simulink model "NLGuidance_12B_with_contracts_PP"  (R2019b)
settings: Solver=FixedStepDiscrete  StartTime=0.0  StopTime=10.0  FixedStep=0.020000  RelTol=1e-3  EnableMultiTasking=on
model workspace (MAT data in the model file):
  ContractValidatorBlocksMap = containers.Map
  ContractValidatorBlocksMap.serialization.keys = {'NLGuidance_12B/contract/validator', 'NLGuidance_12B_with_contracts/contract/validator'}
  ContractValidatorBlocksMap.serialization.values{1}.block = 'NLGuidance_12B/contract/validator'
  ContractValidatorBlocksMap.serialization.values{1}.assumePorts = 2
  ContractValidatorBlocksMap.serialization.values{1}.guaranteePorts = 6
  ContractValidatorBlocksMap.serialization.values{1}.modeBlocksPorts = 0
  ContractValidatorBlocksMap.serialization.values{1}.portHandles.Inport = [1044.00036621 1045.00036621 1046.00036621 1047.00036621 1048.00036621 1049.00036621 1050.00036621 1051.00036621]
  ContractValidatorBlocksMap.serialization.values{1}.portHandles.Outport = 1052.00036621
  ContractValidatorBlocksMap.serialization.values{1}.portHandles.Enable = []
  ContractValidatorBlocksMap.serialization.values{1}.portHandles.Trigger = []
  ContractValidatorBlocksMap.serialization.values{1}.portHandles.State = []
  ContractValidatorBlocksMap.serialization.values{1}.portHandles.LConn = []
  ContractValidatorBlocksMap.serialization.values{1}.portHandles.RConn = []
  ContractValidatorBlocksMap.serialization.values{1}.portHandles.Ifaction = []
  ContractValidatorBlocksMap.serialization.values{1}.portHandles.Reset = []
  ContractValidatorBlocksMap.serialization.values{1}.portConnectivity(1).Type = '1'
  ContractValidatorBlocksMap.serialization.values{1}.portConnectivity(1).Position = [365 -130]
  ContractValidatorBlocksMap.serialization.values{1}.portConnectivity(1).SrcBlock = 945.000488281
  ContractValidatorBlocksMap.serialization.values{1}.portConnectivity(1).SrcPort = 0
  ContractValidatorBlocksMap.serialization.values{1}.portConnectivity(1).DstBlock = []
  ContractValidatorBlocksMap.serialization.values{1}.portConnectivity(1).DstPort = []
  ContractValidatorBlocksMap.serialization.values{1}.portConnectivity(2).Type = '2'
  ContractValidatorBlocksMap.serialization.values{1}.portConnectivity(2).Position = [365 -40]
  ContractValidatorBlocksMap.serialization.values{1}.portConnectivity(2).SrcBlock = 953.000488281
  ContractValidatorBlocksMap.serialization.values{1}.portConnectivity(2).SrcPort = 0
  ContractValidatorBlocksMap.serialization.values{1}.portConnectivity(2).DstBlock = []
  ContractValidatorBlocksMap.serialization.values{1}.portConnectivity(2).DstPort = []
  ContractValidatorBlocksMap.serialization.values{1}.portConnectivity(3).Type = '3'
  ContractValidatorBlocksMap.serialization.values{1}.portConnectivity(3).Position = [365 50]
  ContractValidatorBlocksMap.serialization.values{1}.portConnectivity(3).SrcBlock = 932.000488281
  ContractValidatorBlocksMap.serialization.values{1}.portConnectivity(3).SrcPort = 0
  ContractValidatorBlocksMap.serialization.values{1}.portConnectivity(3).DstBlock = []
  ContractValidatorBlocksMap.serialization.values{1}.portConnectivity(3).DstPort = []
  ContractValidatorBlocksMap.serialization.values{1}.portConnectivity(4).Type = '4'
  ContractValidatorBlocksMap.serialization.values{1}.portConnectivity(4).Position = [365 140]
  ContractValidatorBlocksMap.serialization.values{1}.portConnectivity(4).SrcBlock = 766.000488281
  ContractValidatorBlocksMap.serialization.values{1}.portConnectivity(4).SrcPort = 0
  ContractValidatorBlocksMap.serialization.values{1}.portConnectivity(4).DstBlock = []
  ContractValidatorBlocksMap.serialization.values{1}.portConnectivity(4).DstPort = []
  ContractValidatorBlocksMap.serialization.values{1}.portConnectivity(5).Type = '5'
  ContractValidatorBlocksMap.serialization.values{1}.portConnectivity(5).Position = [365 230]
  ContractValidatorBlocksMap.serialization.values{1}.portConnectivity(5).SrcBlock = 803.000732422
  ContractValidatorBlocksMap.serialization.values{1}.portConnectivity(5).SrcPort = 0
  ContractValidatorBlocksMap.serialization.values{1}.portConnectivity(5).DstBlock = []
  ContractValidatorBlocksMap.serialization.values{1}.portConnectivity(5).DstPort = []
  ContractValidatorBlocksMap.serialization.values{1}.portConnectivity(6).Type = '6'
  ContractValidatorBlocksMap.serialization.values{1}.portConnectivity(6).Position = [365 320]
  ContractValidatorBlocksMap.serialization.values{1}.portConnectivity(6).SrcBlock = 813.000732422
  ContractValidatorBlocksMap.serialization.values{1}.portConnectivity(6).SrcPort = 0
  ContractValidatorBlocksMap.serialization.values{1}.portConnectivity(6).DstBlock = []
  ContractValidatorBlocksMap.serialization.values{1}.portConnectivity(6).DstPort = []
  ContractValidatorBlocksMap.serialization.values{1}.portConnectivity(7).Type = '7'
  ContractValidatorBlocksMap.serialization.values{1}.portConnectivity(7).Position = [365 410]
  ContractValidatorBlocksMap.serialization.values{1}.portConnectivity(7).SrcBlock = 874.000732422
  ContractValidatorBlocksMap.serialization.values{1}.portConnectivity(7).SrcPort = 0
  ContractValidatorBlocksMap.serialization.values{1}.portConnectivity(7).DstBlock = []
  ContractValidatorBlocksMap.serialization.values{1}.portConnectivity(7).DstPort = []
  ContractValidatorBlocksMap.serialization.values{1}.portConnectivity(8).Type = '8'
  ContractValidatorBlocksMap.serialization.values{1}.portConnectivity(8).Position = [365 500]
  ContractValidatorBlocksMap.serialization.values{1}.portConnectivity(8).SrcBlock = 920.000732422
  ContractValidatorBlocksMap.serialization.values{1}.portConnectivity(8).SrcPort = 0
  ContractValidatorBlocksMap.serialization.values{1}.portConnectivity(8).DstBlock = []
  ContractValidatorBlocksMap.serialization.values{1}.portConnectivity(8).DstPort = []
  ContractValidatorBlocksMap.serialization.values{1}.portConnectivity(9).Type = '1'
  ContractValidatorBlocksMap.serialization.values{1}.portConnectivity(9).Position = [510 185]
  ContractValidatorBlocksMap.serialization.values{1}.portConnectivity(9).SrcBlock = []
  ContractValidatorBlocksMap.serialization.values{1}.portConnectivity(9).SrcPort = []
  ContractValidatorBlocksMap.serialization.values{1}.portConnectivity(9).DstBlock = 962.000488281
  ContractValidatorBlocksMap.serialization.values{1}.portConnectivity(9).DstPort = 0
  ContractValidatorBlocksMap.serialization.values{2}.block = 'NLGuidance_12B_with_contracts/contract/validator'
  ContractValidatorBlocksMap.serialization.values{2}.assumePorts = 2
  ContractValidatorBlocksMap.serialization.values{2}.guaranteePorts = 6
  ContractValidatorBlocksMap.serialization.values{2}.modeBlocksPorts = 0
  ContractValidatorBlocksMap.serialization.values{2}.portHandles.Inport = [1044.00183105 1045.00183105 1046.00183105 1047.00183105 1048.00183105 1049.00183105 1050.00183105 1051.00183105]
  ContractValidatorBlocksMap.serialization.values{2}.portHandles.Outport = 1052.00183105
  ContractValidatorBlocksMap.serialization.values{2}.portHandles.Enable = []
  ContractValidatorBlocksMap.serialization.values{2}.portHandles.Trigger = []
  ContractValidatorBlocksMap.serialization.values{2}.portHandles.State = []
  ContractValidatorBlocksMap.serialization.values{2}.portHandles.LConn = []
  ContractValidatorBlocksMap.serialization.values{2}.portHandles.RConn = []
  ContractValidatorBlocksMap.serialization.values{2}.portHandles.Ifaction = []
  ContractValidatorBlocksMap.serialization.values{2}.portHandles.Reset = []
  ContractValidatorBlocksMap.serialization.values{2}.portConnectivity(1).Type = '1'
  ContractValidatorBlocksMap.serialization.values{2}.portConnectivity(1).Position = [365 -130]
  ContractValidatorBlocksMap.serialization.values{2}.portConnectivity(1).SrcBlock = 945.002075195
  ContractValidatorBlocksMap.serialization.values{2}.portConnectivity(1).SrcPort = 0
  ContractValidatorBlocksMap.serialization.values{2}.portConnectivity(1).DstBlock = []
  ContractValidatorBlocksMap.serialization.values{2}.portConnectivity(1).DstPort = []
  ContractValidatorBlocksMap.serialization.values{2}.portConnectivity(2).Type = '2'
  ContractValidatorBlocksMap.serialization.values{2}.portConnectivity(2).Position = [365 -40]
  ContractValidatorBlocksMap.serialization.values{2}.portConnectivity(2).SrcBlock = 953.002075195
  ContractValidatorBlocksMap.serialization.values{2}.portConnectivity(2).SrcPort = 0
  ContractValidatorBlocksMap.serialization.values{2}.portConnectivity(2).DstBlock = []
  ContractValidatorBlocksMap.serialization.values{2}.portConnectivity(2).DstPort = []
  ContractValidatorBlocksMap.serialization.values{2}.portConnectivity(3).Type = '3'
  ContractValidatorBlocksMap.serialization.values{2}.portConnectivity(3).Position = [365 50]
  ContractValidatorBlocksMap.serialization.values{2}.portConnectivity(3).SrcBlock = 932.002075195
  ContractValidatorBlocksMap.serialization.values{2}.portConnectivity(3).SrcPort = 0
  ContractValidatorBlocksMap.serialization.values{2}.portConnectivity(3).DstBlock = []
  ContractValidatorBlocksMap.serialization.values{2}.portConnectivity(3).DstPort = []
  ContractValidatorBlocksMap.serialization.values{2}.portConnectivity(4).Type = '4'
  ContractValidatorBlocksMap.serialization.values{2}.portConnectivity(4).Position = [365 140]
  ContractValidatorBlocksMap.serialization.values{2}.portConnectivity(4).SrcBlock = 766.002075195
  ContractValidatorBlocksMap.serialization.values{2}.portConnectivity(4).SrcPort = 0
  ContractValidatorBlocksMap.serialization.values{2}.portConnectivity(4).DstBlock = []
  ContractValidatorBlocksMap.serialization.values{2}.portConnectivity(4).DstPort = []
  ContractValidatorBlocksMap.serialization.values{2}.portConnectivity(5).Type = '5'
  ContractValidatorBlocksMap.serialization.values{2}.portConnectivity(5).Position = [365 230]
  ContractValidatorBlocksMap.serialization.values{2}.portConnectivity(5).SrcBlock = 803.002075195
  ContractValidatorBlocksMap.serialization.values{2}.portConnectivity(5).SrcPort = 0
  ContractValidatorBlocksMap.serialization.values{2}.portConnectivity(5).DstBlock = []
  ContractValidatorBlocksMap.serialization.values{2}.portConnectivity(5).DstPort = []
  ContractValidatorBlocksMap.serialization.values{2}.portConnectivity(6).Type = '6'
  ContractValidatorBlocksMap.serialization.values{2}.portConnectivity(6).Position = [365 320]
  ContractValidatorBlocksMap.serialization.values{2}.portConnectivity(6).SrcBlock = 813.002075195
  ContractValidatorBlocksMap.serialization.values{2}.portConnectivity(6).SrcPort = 0
  ContractValidatorBlocksMap.serialization.values{2}.portConnectivity(6).DstBlock = []
  ContractValidatorBlocksMap.serialization.values{2}.portConnectivity(6).DstPort = []
  ContractValidatorBlocksMap.serialization.values{2}.portConnectivity(7).Type = '7'
  ContractValidatorBlocksMap.serialization.values{2}.portConnectivity(7).Position = [365 410]
  ContractValidatorBlocksMap.serialization.values{2}.portConnectivity(7).SrcBlock = 874.002075195
  ContractValidatorBlocksMap.serialization.values{2}.portConnectivity(7).SrcPort = 0
  ContractValidatorBlocksMap.serialization.values{2}.portConnectivity(7).DstBlock = []
  ContractValidatorBlocksMap.serialization.values{2}.portConnectivity(7).DstPort = []
  ContractValidatorBlocksMap.serialization.values{2}.portConnectivity(8).Type = '8'
  ContractValidatorBlocksMap.serialization.values{2}.portConnectivity(8).Position = [365 500]
  ContractValidatorBlocksMap.serialization.values{2}.portConnectivity(8).SrcBlock = 920.002075195
  ContractValidatorBlocksMap.serialization.values{2}.portConnectivity(8).SrcPort = 0
  ContractValidatorBlocksMap.serialization.values{2}.portConnectivity(8).DstBlock = []
  ContractValidatorBlocksMap.serialization.values{2}.portConnectivity(8).DstPort = []
  ContractValidatorBlocksMap.serialization.values{2}.portConnectivity(9).Type = '1'
  ContractValidatorBlocksMap.serialization.values{2}.portConnectivity(9).Position = [510 185]
  ContractValidatorBlocksMap.serialization.values{2}.portConnectivity(9).SrcBlock = []
  ContractValidatorBlocksMap.serialization.values{2}.portConnectivity(9).SrcPort = []
  ContractValidatorBlocksMap.serialization.values{2}.portConnectivity(9).DstBlock = 962.002075195
  ContractValidatorBlocksMap.serialization.values{2}.portConnectivity(9).DstPort = 0
  ContractValidatorBlocksMap.serialization.uniformity = 0
  ContractValidatorBlocksMap.serialization.keyType = 'char'
  ContractValidatorBlocksMap.serialization.valueType = 'any'
  already_pp = 1
  compositionalMap.analysisNames = {'NLGuidance_12B_with_contracts_PP/NLGuidance'}
  compositionalMap.compositionalOptions = {{''}}
  compositionalMap.selectedOptions = 1
  nodeNameToBlockNameMap : containers.Map (value not decoded)
  verificationResults.analysisResults{1}.top = 'NLGuidance_12B_with_contracts_PP/NLGuidance'
  verificationResults.analysisResults{1}.abstract = ''
  verificationResults.analysisResults{1}.concrete = 'sqrt_lookup_0_10000,sqrt,r_computation_458_001,norm_885_002,norm_827_002,norm_237_001,norm2_847_002,norm2_639_002,norm1_895_002,norm1_837_002,norm1_777_002,norm1_629_002,norm1_247_001,kind2_times,kind2_divide,cross_400_001,assumeXrnotnull_953_002,assumeVvnotnull_945_002,Subsystem2_427_001,Subsystem1_405_001,Outer_316_001_condExecSS,Outer_316_001,NLG_001_932_002,NLG007_920_002,NLG006_874_002,NLG005_813_002,NLG004_803_002,NLG002_NLG003_766_002,Inner_53_001_condExecSS,Inner_53_001,Implies_821_002,DotProduct_807_002,DotProduct_772_002,DotProduct_1148_002,Compare_newline_ToZero_955_002,Compare_newline_ToZero_947_002,Compare_newline_ToZero_935_002,Compare_newline_ToZero_923_002,Compare_newline_ToZero_806_002,Compare_newline_ToZero_771_002,CW_333_001_condExecSS,CW_333_001,CCW_328_001_condExecSS,CCW_328_001,Arg2_139_001,Arg1_70_001,Act2_65_001_condExecSS,Act2_65_001,Act1_60_001_condExecSS,Act1_60_001'
  verificationResults.analysisResults{1}.assumptions = '(NLG002_NLG003_766_002,1)'
  verificationResults.analysisResults{1}.properties{1}.propertyName = 'contract_733_002[l1096c1].NLG002_NLG003_766_002[1]'
  verificationResults.analysisResults{1}.properties{1}.answer = 'UNKNOWN'
  verificationResults.analysisResults{1}.properties{1}.originPath = 'NLGuidance_12B_with_contracts_PP/contract/NLG002_NLG003'
  verificationResults.analysisResults{1}.properties{1}.propertyType = 'guarantee'
  verificationResults.analysisResults{1}.properties{2}.propertyName = 'contract_733_002[l1096c1].NLG004_803_002[2]'
  verificationResults.analysisResults{1}.properties{2}.answer = 'UNKNOWN'
  verificationResults.analysisResults{1}.properties{2}.originPath = 'NLGuidance_12B_with_contracts_PP/contract/NLG004'
  verificationResults.analysisResults{1}.properties{2}.propertyType = 'guarantee'
  verificationResults.analysisResults{1}.properties{3}.propertyName = 'contract_733_002[l1096c1].NLG005_813_002[3]'
  verificationResults.analysisResults{1}.properties{3}.answer = 'UNKNOWN'
  verificationResults.analysisResults{1}.properties{3}.originPath = 'NLGuidance_12B_with_contracts_PP/contract/NLG005'
  verificationResults.analysisResults{1}.properties{3}.propertyType = 'guarantee'
  verificationResults.analysisResults{1}.properties{4}.propertyName = 'contract_733_002[l1096c1].NLG006_874_002[4]'
  verificationResults.analysisResults{1}.properties{4}.answer = 'UNKNOWN'
  verificationResults.analysisResults{1}.properties{4}.originPath = 'NLGuidance_12B_with_contracts_PP/contract/NLG006'
  verificationResults.analysisResults{1}.properties{4}.propertyType = 'guarantee'
  verificationResults.analysisResults{1}.properties{5}.propertyName = 'contract_733_002[l1096c1].NLG007_920_002[5]'
  verificationResults.analysisResults{1}.properties{5}.answer = 'UNKNOWN'
  verificationResults.analysisResults{1}.properties{5}.originPath = 'NLGuidance_12B_with_contracts_PP/contract/NLG007'
  verificationResults.analysisResults{1}.properties{5}.propertyType = 'guarantee'
  verificationResults.analysisResults{1}.properties{6}.propertyName = 'contract_733_002[l1096c1].NLG_001_932_002[6]'
  verificationResults.analysisResults{1}.properties{6}.answer = 'UNKNOWN'
  verificationResults.analysisResults{1}.properties{6}.originPath = 'NLGuidance_12B_with_contracts_PP/contract/NLG_001'
  verificationResults.analysisResults{1}.properties{6}.propertyType = 'guarantee'
  verificationResults.sampleTime = 0.02
undefined symbols (not defined in the file): contractAfterSimulation, ContractAssumeBlock, contractBeforeSimulation, ContractBlock, ContractGuaranteeBlock, ContractValidatorBlock, DotProduct, pp_lib, saveValidatorParameters
settings Model: Creator=elliocm  LastModifiedBy=hbourbou
settings DataIOCC: LimitDataPoints=on  SaveFormat=Array  SignalLoggingSaveFormat=ModelDataLogs  ReturnWorkspaceOutputs=off
settings OptimizationCC: ExpressionDepthLimit=2147483647  LifeSpan=inf
settings DebuggingCC: AlgebraicLoopMsg=error  ArtificialAlgebraicLoopMsg=error  UnderspecifiedInitializationDetection=Classic  MergeDetectMultiDrivingBlocksExec=none  SolverPrmCheckMsg=warning  MultiTaskDSMMsg=warning  MultiTaskCondExecSysMsg=none  SingleTaskRateTransMsg=error  StateNameClashWarn=warning  SFUnexpectedBacktrackingDiag=warning  SFNoUnconditionalDefaultTransitionDiag=warning  SFExecutionAtInitializationDiag=none  ArithmeticOperatorsInVariantConditions=warning
settings HardwareCC: ProdBitPerPointer=32  ProdBitPerSizeT=32  ProdBitPerPtrDiffT=32  ProdLargestAtomicFloat=None  ProdIntDivRoundTo=Undefined  ProdEndianess=Unspecified  ProdWordSize=32  ProdHWDeviceType=32-bit Generic
settings ModelReferenceCC: PropagateSignalLabelsOutOfModel=off
settings SFSimCC: SimUseLocalCustomCode=off  CustomCodeUndefinedFunction=UseInterfaceOnly
settings RTWCC: RTWUseLocalCustomCode=off
settings CodeAppCC: StateflowObjectComments=on
settings GRTTargetCC: TargetLangStandard=C89/C90 (ANSI)  GeneratePreprocessorConditionals=Disable all
settings ConfigComp: CovMetricSettings=dw  CovHtmlReporting=on  CovSaveCumulativeToWorkspaceVar=on  CovSaveSingleToWorkspaceVar=on  CovExternalEMLEnable=off  DVMode=PropertyProving  DVMaxProcessTime=7200  DVTestSuiteOptimization=CombinedObjectives (Nonlinear Extended)

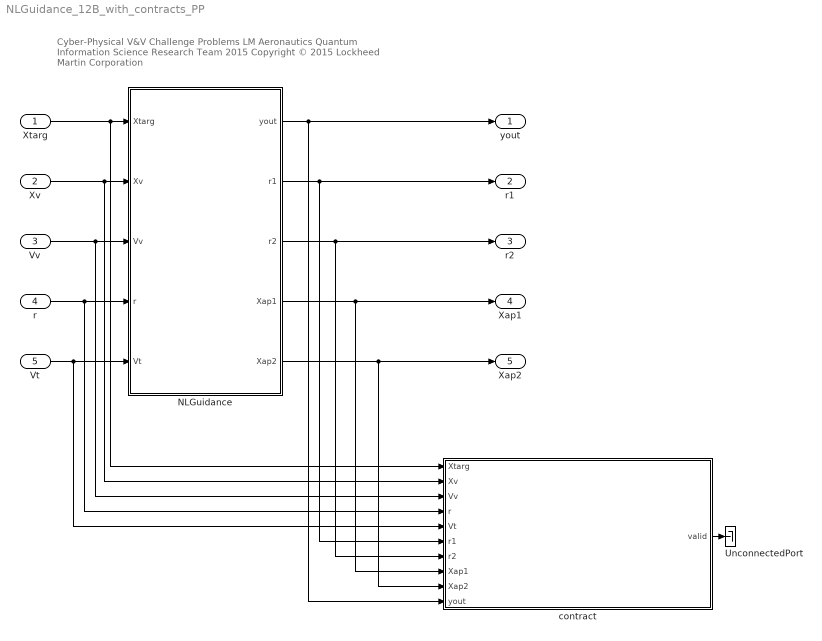
== system NLGuidance_12B_with_contracts_PP ==
  note: Cyber-Physical V&V Challenge Problems
      | LM Aeronautics Quantum Information Science Research Team 2015
      | Copyright © 2015 Lockheed Martin Corporation
  Xtarg : Inport  OutDataTypeStr=double  PortDimensions=3
  Xv : Inport  Port=2  OutDataTypeStr=double  PortDimensions=3
  Vv : Inport  Port=3  OutDataTypeStr=double  PortDimensions=3
  r : Inport  Port=4  OutDataTypeStr=double
  Vt : Inport  Port=5  OutDataTypeStr=double  PortDimensions=3
  NLGuidance : Subsystem  TreatAsAtomicUnit=on
  UnconnectedPort : Terminator
  contract : Subsystem  TreatAsAtomicUnit=on  mask(ContractBlock){ContractBlockType=ContractBlock}
      mask init:
      | set_param(gcb, 'LinkStatus', 'none');
      settings: CopyFcn=set_param(gcb, 'LinkStatus', 'none');
      mask DialogControl DescTextVar Prompt: Contract block
      mask Display:
      | text(0.5, 0.5, '{\bf\fontsize{20}Contract}', 'hor', 'center', 'texmode','on');
      | blocks = find_system(gcb, 'LookUnderMasks','all', 'SearchDepth',1,'BlockType','Inport');
      | for i = 1 : length(blocks)
      |     blockName = get_param(blocks(i), 'Name');
      |     [path, blockName] = fileparts(char(blockName));
      |     port_label('input', i, blockName);
      | end
      | 
      | blocks = find_system(gcb, 'LookUnderMasks','all', 'SearchDepth',1,'BlockType','Outport');
      | for i = 1 : length(blocks)
      |     blockName = get_param(blocks(i), 'Name');
      |     [path, blockName] = fileparts(char(blockName));
      |     port_label('output', i, blockName);
      | end
  yout : Outport  VectorParamsAs1DForOutWhenUnconnected=off
  r1 : Outport  Port=2  VectorParamsAs1DForOutWhenUnconnected=off
  r2 : Outport  Port=3  VectorParamsAs1DForOutWhenUnconnected=off
  Xap1 : Outport  Port=4  VectorParamsAs1DForOutWhenUnconnected=off
  Xap2 : Outport  Port=5  VectorParamsAs1DForOutWhenUnconnected=off
  wires:
  NLGuidance/1(yout) -> contract/10(yout), yout/1
  Xv/1 -> contract/2(Xv), NLGuidance/2(Xv)
  Vv/1 -> contract/3(Vv), NLGuidance/3(Vv)
  r/1 -> contract/4(r), NLGuidance/4(r)
  Vt/1 -> contract/5(Vt), NLGuidance/5(Vt)
  Xtarg/1 -> contract/1(Xtarg), NLGuidance/1(Xtarg)
  NLGuidance/3(r2) -> contract/7(r2), r2/1
  NLGuidance/4(Xap1) -> contract/8(Xap1), Xap1/1
  NLGuidance/5(Xap2) -> contract/9(Xap2), Xap2/1
  NLGuidance/2(r1) -> contract/6(r1), r1/1
  contract/1(valid) -> UnconnectedPort/1

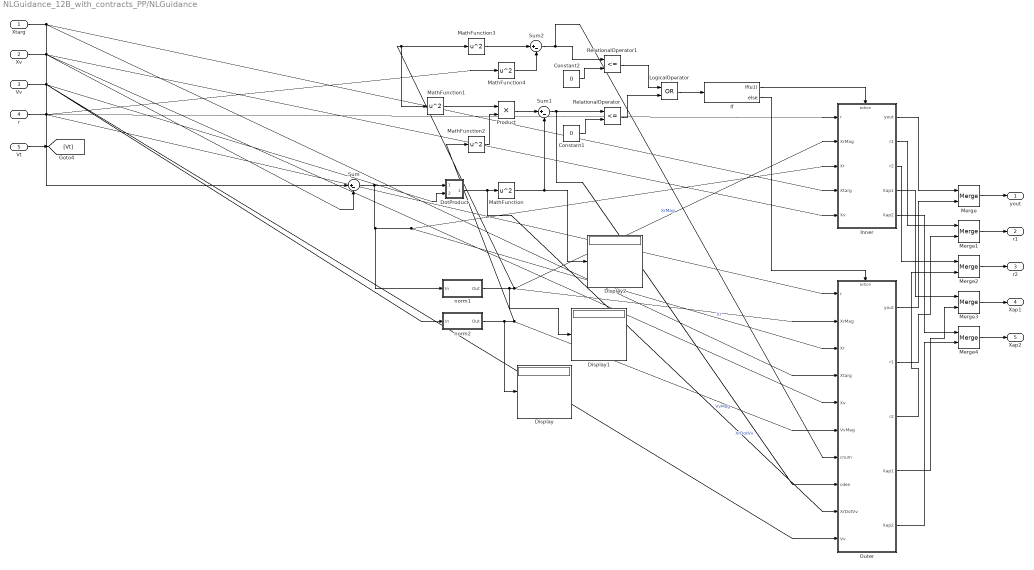
== system NLGuidance_12B_with_contracts_PP/NLGuidance ==
  Xtarg : Inport
  Xv : Inport  Port=2
  Vv : Inport  Port=3
  r : Inport  Port=4
  Vt : Inport  Port=5
  Constant1 : Constant  Value=0
  Constant2 : Constant  Value=0
  Display : Display
  Display1 : Display
  Display2 : Display
  DotProduct : Subsystem  AncestorBlock=pp_lib/DotProduct  TreatAsAtomicUnit=on
  If : If  IfExpression=u1
  Inner : Subsystem  TreatAsAtomicUnit=on
  LogicalOperator : Logic  Operator=OR  AllPortsSameDT=off  OutDataTypeStr=boolean
  MathFunction{,1..4} (5 alike) : Math  Operator=square  SaturateOnIntegerOverflow=on
  Merge{,1..4} (5 alike) : Merge
  Outer : Subsystem  TreatAsAtomicUnit=on
  Product : Product  RndMeth=Zero
  RelationalOperator : RelationalOperator  Operator=<=  OutDataTypeStr=boolean  RndMeth=Nearest
  RelationalOperator1 : RelationalOperator  Operator=<=  OutDataTypeStr=boolean  RndMeth=Nearest
  Sum : Sum  Inputs=|+-
  Sum1 : Sum  Inputs=|+-
  Sum2 : Sum  Inputs=|+-
  norm1 : Subsystem  TreatAsAtomicUnit=on
  norm2 : Subsystem  TreatAsAtomicUnit=on
  yout : Outport  VectorParamsAs1DForOutWhenUnconnected=off
  r1 : Outport  Port=2  VectorParamsAs1DForOutWhenUnconnected=off
  r2 : Outport  Port=3  VectorParamsAs1DForOutWhenUnconnected=off
  Xap1 : Outport  Port=4  VectorParamsAs1DForOutWhenUnconnected=off
  Xap2 : Outport  Port=5  VectorParamsAs1DForOutWhenUnconnected=off
  wires:
  Vt/1 -> [Vt]
  Xtarg/1 -> Sum/1, Inner/4(Xtarg), Outer/4(Xtarg)
  Sum/1 -> norm1/1(In), Inner/3(Xr), Outer/3(Xr), DotProduct/1(In1)  "Xr"
  DotProduct/1(Out1) -> MathFunction/1, Outer/9(XrDotVv)  "XrDotVv"
  norm1/1(Out) -> Display1/1, Inner/2(XrMag), Outer/2(XrMag), MathFunction1/1, MathFunction3/1  "XrMag"
  norm2/1(Out) -> Display/1, Outer/6(VvMag), MathFunction2/1  "VvMag"
  MathFunction/1 -> Display2/1, Sum1/2
  MathFunction1/1 -> Product/1
  MathFunction2/1 -> Product/2
  Product/1 -> Sum1/1
  Sum1/1 -> RelationalOperator/1, Outer/8(cden)
  Constant1/1 -> RelationalOperator/2
  RelationalOperator/1 -> LogicalOperator/2
  Sum2/1 -> RelationalOperator1/1, Outer/7(cnum)
  Constant2/1 -> RelationalOperator1/2
  RelationalOperator1/1 -> LogicalOperator/1
  MathFunction3/1 -> Sum2/1
  MathFunction4/1 -> Sum2/2
  LogicalOperator/1 -> If/1
  Xv/1 -> Inner/5(Xv), Outer/5(Xv), Sum/2
  Inner/1(yout) -> Merge/1
  Outer/1(yout) -> Merge/2
  If/1 -> Inner/Action
  If/2 -> Outer/Action
  r/1 -> Outer/1(r), MathFunction4/1, Inner/1(r)
  Vv/1 -> Outer/10(Vv), DotProduct/2(In2), norm2/1(In)
  Merge/1 -> yout/1
  Merge1/1 -> r1/1
  Inner/2(r1) -> Merge1/1
  Outer/2(r1) -> Merge1/2
  Merge2/1 -> r2/1
  Outer/3(r2) -> Merge2/2
  Inner/3(r2) -> Merge2/1
  Merge3/1 -> Xap1/1
  Merge4/1 -> Xap2/1
  Inner/4(Xap1) -> Merge3/1
  Outer/4(Xap1) -> Merge3/2
  Inner/5(Xap2) -> Merge4/1
  Outer/5(Xap2) -> Merge4/2

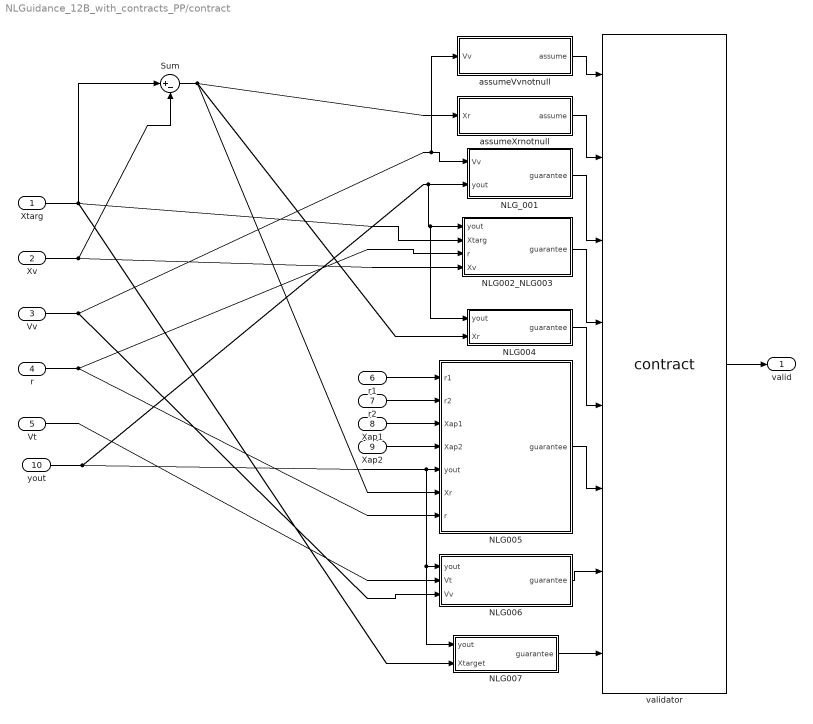
== system NLGuidance_12B_with_contracts_PP/contract ==
  Xtarg : Inport  OutDataTypeStr=double  PortDimensions=3
  Xv : Inport  Port=2  OutDataTypeStr=double  PortDimensions=3
  Vv : Inport  Port=3  OutDataTypeStr=double  PortDimensions=3
  r : Inport  Port=4  OutDataTypeStr=double
  Vt : Inport  Port=5  OutDataTypeStr=double  PortDimensions=3
  r1 : Inport  Port=6
  r2 : Inport  Port=7
  Xap1 : Inport  Port=8
  Xap2 : Inport  Port=9
  yout : Inport  Port=10
  NLG002_NLG003 : Subsystem  TreatAsAtomicUnit=on  mask(ContractGuaranteeBlock){ContractBlockType=ContractGuaranteeBlock}
      mask init:
      | set_param(gcb, 'LinkStatus', 'none');
      mask DialogControl DescTextVar Prompt: Guarantee block
  NLG004 : Subsystem  TreatAsAtomicUnit=on  mask(ContractGuaranteeBlock){ContractBlockType=ContractGuaranteeBlock}
      mask init:
      | set_param(gcb, 'LinkStatus', 'none');
      mask DialogControl DescTextVar Prompt: Guarantee block
  NLG005 : Subsystem  TreatAsAtomicUnit=on  mask(ContractGuaranteeBlock){ContractBlockType=ContractGuaranteeBlock}
      mask init:
      | set_param(gcb, 'LinkStatus', 'none');
      mask DialogControl DescTextVar Prompt: Guarantee block
  NLG006 : Subsystem  TreatAsAtomicUnit=on  mask(ContractGuaranteeBlock){ContractBlockType=ContractGuaranteeBlock}
      mask init:
      | set_param(gcb, 'LinkStatus', 'none');
      mask DialogControl DescTextVar Prompt: Guarantee block
  NLG007 : Subsystem  TreatAsAtomicUnit=on  mask(ContractGuaranteeBlock){ContractBlockType=ContractGuaranteeBlock}
      mask init:
      | set_param(gcb, 'LinkStatus', 'none');
      mask DialogControl DescTextVar Prompt: Guarantee block
  NLG_001 : Subsystem  TreatAsAtomicUnit=on  mask(ContractGuaranteeBlock){ContractBlockType=ContractGuaranteeBlock}
      mask init:
      | set_param(gcb, 'LinkStatus', 'none');
      mask DialogControl DescTextVar Prompt: Guarantee block
  Sum : Sum  Inputs=|+-
  assumeVvnotnull : Subsystem  TreatAsAtomicUnit=on  mask(ContractAssumeBlock){ContractBlockType=ContractAssumeBlock}
      mask init:
      | set_param(gcb, 'LinkStatus', 'none');
      mask DialogControl DescTextVar Prompt: Assume block
  assumeXrnotnull : Subsystem  TreatAsAtomicUnit=on  mask(ContractAssumeBlock){ContractBlockType=ContractAssumeBlock}
      mask init:
      | set_param(gcb, 'LinkStatus', 'none');
      mask DialogControl DescTextVar Prompt: Assume block
  validator : M-S-Function  LoadFcn=saveValidatorParameters(gcb);  InitFcn=contractBeforeSimulation();  StopFcn=contractAfterSimulation();  FunctionName=contract  mask(ContractValidatorBlock){assumePorts=2, guaranteePorts=6, modePorts=0, ContractBlockType=ContractValidatorBlock, createInportsCheckbox=off}
      mask prompts: assumePorts "Assume ports     :"; guaranteePorts "Guarantee ports :"; modePorts "Mode ports        :"; createInportsCheckbox "Create inports and connect them automatically"
      mask init:
      | set_param(gcb,'LinkStatus','none');
      | contract_callback('inputs_callback',gcb);
      mask DialogControl DescTextVar Prompt: The validator block implements the following logic: <br> <br> <b>Sofar</b>(assume<sub>1</sub> <b>&#8743;</b> assume<sub>2</sub> <b>&#8743;</b> ... assume<sub>k</sub>) <b>&rarr;</b> (guarantee<sub>1</sub> <b>&#8743;</b> guarantee<sub>2</sub> <b>&#8743;</b> ... guarantee<sub>m</sub> <b>&#8743;</b>  mode<sub>1</sub> <b>&#8743;</b> mode<sub>2</sub> <b>&#8743;</b> ... <b>&#8743;</b> mode<sub>n</sub> )<br> where mode<sub>i</sub> = require<sub>i</sub> <b>&rarr;</b> ensure<sub>i</sub>
      mask Display:
      | color('black');
      | port_label('input',1,'assume');
      | port_label('input',2,'assume');
      | port_label('input',3,'guarantee');
      | port_label('input',4,'guarantee');
      | port_label('input',5,'guarantee');
      | port_label('input',6,'guarantee');
      | port_label('input',7,'guarantee');
      | port_label('input',8,'guarantee');
      | port_label('output',1,'valid');
  valid : Outport  VectorParamsAs1DForOutWhenUnconnected=off
  wires:
  validator/1 -> valid/1
  Xv/1 -> Sum/2, NLG002_NLG003/4(Xv)
  Xtarg/1 -> Sum/1, NLG007/2(Xtarget), NLG002_NLG003/2(Xtarg)
  yout/1 -> NLG004/1(yout), NLG002_NLG003/1(yout), NLG_001/2(yout), NLG007/1(yout), NLG006/1(yout), NLG005/5(yout)
  NLG_001/1(guarantee) -> validator/3
  NLG002_NLG003/1(guarantee) -> validator/4
  NLG004/1(guarantee) -> validator/5
  NLG005/1(guarantee) -> validator/6
  NLG006/1(guarantee) -> validator/7
  NLG007/1(guarantee) -> validator/8
  assumeVvnotnull/1(assume) -> validator/1
  assumeXrnotnull/1(assume) -> validator/2
  r1/1 -> NLG005/1(r1)
  r2/1 -> NLG005/2(r2)
  Xap1/1 -> NLG005/3(Xap1)
  Xap2/1 -> NLG005/4(Xap2)
  Sum/1 -> NLG005/6(Xr), assumeXrnotnull/1(Xr), NLG004/2(Xr)
  r/1 -> NLG005/7(r), NLG002_NLG003/3(r)
  Vt/1 -> NLG006/2(Vt)
  Vv/1 -> NLG006/3(Vv), assumeVvnotnull/1(Vv), NLG_001/1(Vv)

== system NLGuidance_12B_with_contracts_PP/NLGuidance/DotProduct ==
  In1 : Inport
  In2 : Inport  Port=2
  Product : Product  InputSameDT=on
  SSpec1 : SignalSpecification  Dimensions=3
  SSpec2 : SignalSpecification  Dimensions=3
  Sum : Sum  Inputs=1
  Out1 : Outport  VectorParamsAs1DForOutWhenUnconnected=off
  wires:
  SSpec2/1 -> Product/2
  SSpec1/1 -> Product/1
  Sum/1 -> Out1/1
  Product/1 -> Sum/1
  In1/1 -> SSpec1/1
  In2/1 -> SSpec2/1

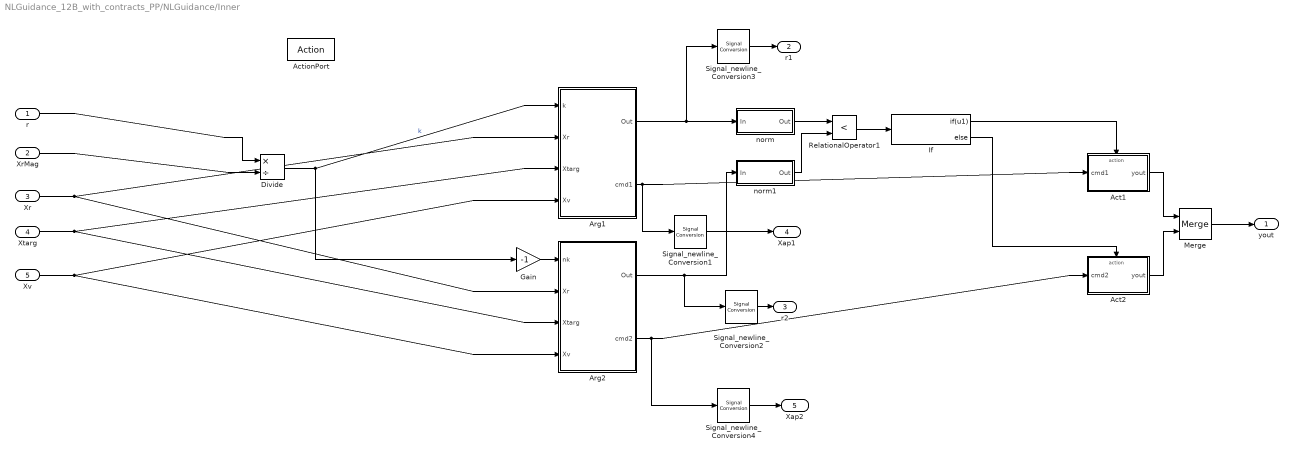
== system NLGuidance_12B_with_contracts_PP/NLGuidance/Inner ==
  r : Inport
  XrMag : Inport  Port=2
  Xr : Inport  Port=3
  Xtarg : Inport  Port=4
  Xv : Inport  Port=5
  ActionPort : ActionPort  ActionPortLabel=if(u1)
  Act1 : Subsystem  TreatAsAtomicUnit=on
  Act2 : Subsystem  TreatAsAtomicUnit=on
  Arg1 : Subsystem  TreatAsAtomicUnit=on
  Arg2 : Subsystem  TreatAsAtomicUnit=on
  Divide : Product  Inputs=*/
  Gain : Gain  Gain=-1
  If : If  IfExpression=u1
  Merge : Merge
  RelationalOperator1 : RelationalOperator  Operator=<  OutDataTypeStr=boolean  RndMeth=Nearest
  Signal_newline_Conversion{1..4} (4 alike) : SignalConversion  OverrideOpt=off
  norm : Subsystem  TreatAsAtomicUnit=on
  norm1 : Subsystem  TreatAsAtomicUnit=on
  yout : Outport  VectorParamsAs1DForOutWhenUnconnected=off
  r1 : Outport  Port=2  VectorParamsAs1DForOutWhenUnconnected=off
  r2 : Outport  Port=3  VectorParamsAs1DForOutWhenUnconnected=off
  Xap1 : Outport  Port=4  VectorParamsAs1DForOutWhenUnconnected=off
  Xap2 : Outport  Port=5  VectorParamsAs1DForOutWhenUnconnected=off
  wires:
  r/1 -> Divide/1
  XrMag/1 -> Divide/2
  norm/1(Out) -> RelationalOperator1/1
  norm1/1(Out) -> RelationalOperator1/2
  Arg1/1(Out) -> Signal_newline_Conversion3/1, norm/1(In)
  Divide/1 -> Arg1/1(k), Gain/1  "k"
  Xr/1 -> Arg1/2(Xr), Arg2/2(Xr)
  RelationalOperator1/1 -> If/1
  Xtarg/1 -> Arg2/3(Xtarg), Arg1/3(Xtarg)
  Xv/1 -> Arg2/4(Xv), Arg1/4(Xv)
  Arg2/1(Out) -> Signal_newline_Conversion2/1, norm1/1(In)
  Gain/1 -> Arg2/1(nk)
  Arg1/2(cmd1) -> Signal_newline_Conversion1/1, Act1/1(cmd1)
  Act1/1(yout) -> Merge/1
  Act2/1(yout) -> Merge/2
  Merge/1 -> yout/1
  If/1 -> Act1/Action
  If/2 -> Act2/Action
  Arg2/2(cmd2) -> Signal_newline_Conversion4/1, Act2/1(cmd2)
  Signal_newline_Conversion3/1 -> r1/1
  Signal_newline_Conversion1/1 -> Xap1/1
  Signal_newline_Conversion2/1 -> r2/1
  Signal_newline_Conversion4/1 -> Xap2/1

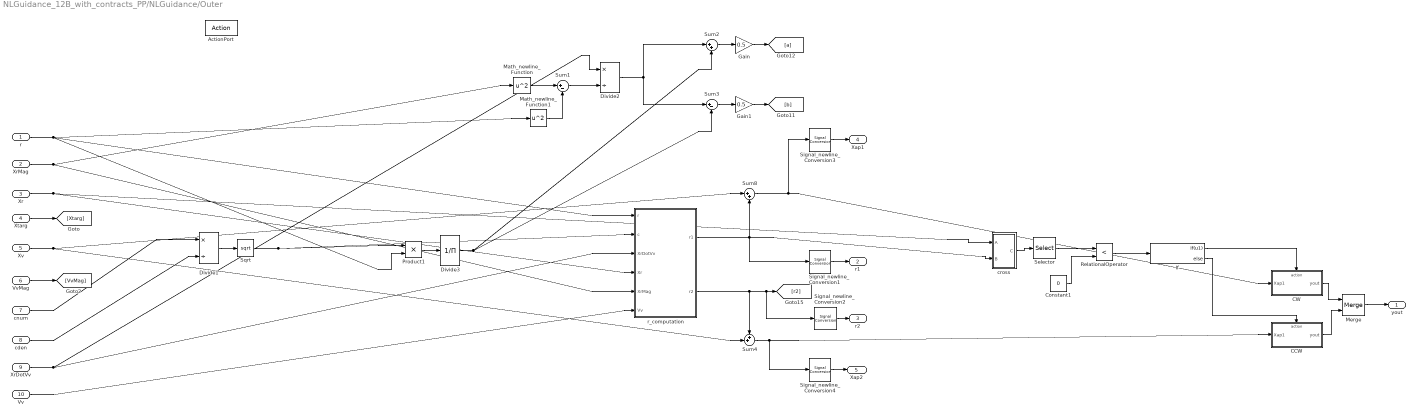
== system NLGuidance_12B_with_contracts_PP/NLGuidance/Outer ==
  r : Inport
  XrMag : Inport  Port=2
  Xr : Inport  Port=3
  Xtarg : Inport  Port=4
  Xv : Inport  Port=5
  VvMag : Inport  Port=6
  cnum : Inport  Port=7
  cden : Inport  Port=8
  XrDotVv : Inport  Port=9
  Vv : Inport  Port=10
  ActionPort : ActionPort  ActionPortLabel=else
  CCW : Subsystem  TreatAsAtomicUnit=on
  CW : Subsystem  TreatAsAtomicUnit=on
  Constant1 : Constant  Value=0
  Divide1 : Product  Inputs=*/
  Divide2 : Product  Inputs=*/
  Divide3 : Product  Inputs=/
  Gain : Gain  Gain=0.5
  Gain1 : Gain  Gain=0.5
  If : If  IfExpression=u1
  Math_newline_Function : Math  Operator=square  SaturateOnIntegerOverflow=on
  Math_newline_Function1 : Math  Operator=square  SaturateOnIntegerOverflow=on
  Merge : Merge
  Product1 : Product
  RelationalOperator : RelationalOperator  Operator=<  OutDataTypeStr=boolean  RndMeth=Nearest
  Selector : Selector  InputPortWidth=3  IndexOptions=Index vector (dialog)  Indices=[3]  OutputSizes=1
  Signal_newline_Conversion{1..4} (4 alike) : SignalConversion  OverrideOpt=off
  Sqrt : Sqrt  SaturateOnIntegerOverflow=on
  Sum1 : Sum  Inputs=|+-
  Sum2 : Sum  Inputs=|++
  Sum3 : Sum  Inputs=|+-
  Sum4 : Sum  Inputs=++|
  Sum8 : Sum  Inputs=|++
  cross : Subsystem  TreatAsAtomicUnit=on
  r_computation : Subsystem  TreatAsAtomicUnit=on
  yout : Outport  VectorParamsAs1DForOutWhenUnconnected=off
  r1 : Outport  Port=2  VectorParamsAs1DForOutWhenUnconnected=off
  r2 : Outport  Port=3  VectorParamsAs1DForOutWhenUnconnected=off
  Xap1 : Outport  Port=4  VectorParamsAs1DForOutWhenUnconnected=off
  Xap2 : Outport  Port=5  VectorParamsAs1DForOutWhenUnconnected=off
  wires:
  Xtarg/1 -> [Xtarg]
  r/1 -> Math_newline_Function1/1, Product1/2, r_computation/1(r)
  VvMag/1 -> [VvMag]
  cnum/1 -> Divide1/1
  cden/1 -> Divide1/2
  Divide1/1 -> Sqrt/1
  Math_newline_Function/1 -> Sum1/1
  Math_newline_Function1/1 -> Sum1/2
  Sum1/1 -> Divide2/2
  Divide2/1 -> Sum3/1, Sum2/1
  Sum2/1 -> Gain/1
  Sum3/1 -> Gain1/1
  Product1/1 -> Divide3/1
  Divide3/1 -> Sum3/2, Sum2/2
  Gain1/1 -> [b]
  Gain/1 -> [a]
  r_computation/1(r1) -> Signal_newline_Conversion1/1, Sum8/2, cross/2(B)
  r_computation/2(r2) -> Sum4/1, Signal_newline_Conversion2/1, [r2]
  Xv/1 -> Sum8/1, Sum4/2
  Sum8/1 -> Signal_newline_Conversion3/1, CW/1(Xap1)
  Sum4/1 -> Signal_newline_Conversion4/1, CCW/1(Xap1)
  Sqrt/1 -> r_computation/2(c), Product1/1
  XrDotVv/1 -> r_computation/3(XrDotVv), Divide2/1
  Xr/1 -> r_computation/4(Xr), cross/1(A)
  XrMag/1 -> r_computation/5(XrMag), Math_newline_Function/1
  Vv/1 -> r_computation/6(Vv)
  cross/1(C) -> Selector/1
  Constant1/1 -> RelationalOperator/2
  Selector/1 -> RelationalOperator/1
  RelationalOperator/1 -> If/1
  If/1 -> CW/Action
  If/2 -> CCW/Action
  CW/1(yout) -> Merge/1
  CCW/1(yout) -> Merge/2
  Merge/1 -> yout/1
  Signal_newline_Conversion3/1 -> Xap1/1
  Signal_newline_Conversion1/1 -> r1/1
  Signal_newline_Conversion2/1 -> r2/1
  Signal_newline_Conversion4/1 -> Xap2/1

== system NLGuidance_12B_with_contracts_PP/NLGuidance/norm1 ==
  In : Inport
  Math_newline_Function : Math  Operator=square  SaturateOnIntegerOverflow=on
  Math_newline_Function1 : Math  Operator=sqrt  SaturateOnIntegerOverflow=on
  Sumof_newline_Elements : Sum  Inputs=+
  Out : Outport  VectorParamsAs1DForOutWhenUnconnected=off
  wires:
  Math_newline_Function/1 -> Sumof_newline_Elements/1
  Sumof_newline_Elements/1 -> Math_newline_Function1/1
  In/1 -> Math_newline_Function/1
  Math_newline_Function1/1 -> Out/1

== system NLGuidance_12B_with_contracts_PP/NLGuidance/norm2 ==
  In : Inport
  Math_newline_Function : Math  Operator=square  SaturateOnIntegerOverflow=on
  Math_newline_Function1 : Math  Operator=sqrt  SaturateOnIntegerOverflow=on
  Sumof_newline_Elements : Sum  Inputs=+
  Out : Outport  VectorParamsAs1DForOutWhenUnconnected=off
  wires:
  Math_newline_Function1/1 -> Out/1
  In/1 -> Math_newline_Function/1
  Sumof_newline_Elements/1 -> Math_newline_Function1/1
  Math_newline_Function/1 -> Sumof_newline_Elements/1

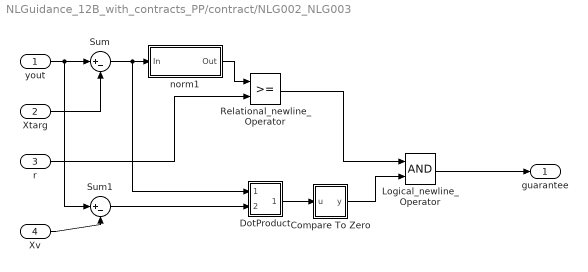
== system NLGuidance_12B_with_contracts_PP/contract/NLG002_NLG003 ==
  yout : Inport
  Xtarg : Inport  Port=2
  r : Inport  Port=3
  Xv : Inport  Port=4
  Compare To Zero : Subsystem  AncestorBlock=|  TreatAsAtomicUnit=on  mask(Compare To Zero){relop===, OutDataTypeStr=boolean, ZeroCross=on}
      | simulink/Logic and Bit
      | Operations/Compare
      | To Zero
      mask prompts: relop "Simulink:masks:Operator_MP"; OutDataTypeStr "Simulink:masks:OutputDataType_MP"; ZeroCross "Simulink:masks:EnableZerocrossingDetection_MP"
      mask help: Simulink:masks:CompareToZero_MD
      mask init:
      | blkName = gcb;
      | 
      | if strcmp(get_param(gcbh,'OutDataTypeStr'),'boolean')
      | 	setValue = 'boolean';
      | else
      |     setValue = 'fixdt(0, 8)';
      | end
      | 
      | set_param([blkName,'/Compare'],'relop',relop, ...
      | 	'OutDataTypeStr', setValue, 'ZeroCross', ZeroCross);
      mask TypeOptions relop: == | ~= | < | <= | >= | >
      mask TypeOptions OutDataTypeStr: Simulink:masks:uint8 | Simulink:masks:boolean
      mask Callback ZeroCross: sl('zeroCrossEnable', gcbh);
      mask Display: disp([relop,' 0'])
  DotProduct : Subsystem  AncestorBlock=pp_lib/DotProduct  TreatAsAtomicUnit=on
  Logical_newline_Operator : Logic  AllPortsSameDT=off  OutDataTypeStr=boolean
  Relational_newline_Operator : RelationalOperator  OutDataTypeStr=boolean  RndMeth=Simplest
  Sum : Sum  Inputs=|+-
  Sum1 : Sum  Inputs=|+-
  norm1 : Subsystem  TreatAsAtomicUnit=on
  guarantee : Outport  OutDataTypeStr=boolean  VectorParamsAs1DForOutWhenUnconnected=off
  wires:
  Logical_newline_Operator/1 -> guarantee/1
  Xtarg/1 -> Sum/2
  yout/1 -> Sum1/1, Sum/1
  Sum/1 -> DotProduct/1(In1), norm1/1(In)
  norm1/1(Out) -> Relational_newline_Operator/1
  r/1 -> Relational_newline_Operator/2
  Relational_newline_Operator/1 -> Logical_newline_Operator/1
  Xv/1 -> Sum1/2
  Sum1/1 -> DotProduct/2(In2)
  DotProduct/1(Out1) -> Compare To Zero/1(u)
  Compare To Zero/1(y) -> Logical_newline_Operator/2

== system NLGuidance_12B_with_contracts_PP/contract/NLG004 ==
  yout : Inport
  Xr : Inport  Port=2
  Compare To Zero : Subsystem  AncestorBlock=|  TreatAsAtomicUnit=on  mask(Compare To Zero){relop=>, OutDataTypeStr=boolean, ZeroCross=on}
      | simulink/Logic and Bit
      | Operations/Compare
      | To Zero
      mask prompts: relop "Simulink:masks:Operator_MP"; OutDataTypeStr "Simulink:masks:OutputDataType_MP"; ZeroCross "Simulink:masks:EnableZerocrossingDetection_MP"
      mask help: Simulink:masks:CompareToZero_MD
      mask init: same as NLGuidance_12B_with_contracts_PP/contract/NLG002_NLG003/Compare To Zero
      mask TypeOptions relop: == | ~= | < | <= | >= | >
      mask TypeOptions OutDataTypeStr: Simulink:masks:uint8 | Simulink:masks:boolean
      mask Callback ZeroCross: sl('zeroCrossEnable', gcbh);
      mask Display: disp([relop,' 0'])
  DotProduct : Subsystem  AncestorBlock=pp_lib/DotProduct  TreatAsAtomicUnit=on
  guarantee : Outport  OutDataTypeStr=boolean  VectorParamsAs1DForOutWhenUnconnected=off
  wires:
  Compare To Zero/1(y) -> guarantee/1
  DotProduct/1(Out1) -> Compare To Zero/1(u)
  yout/1 -> DotProduct/1(In1)
  Xr/1 -> DotProduct/2(In2)

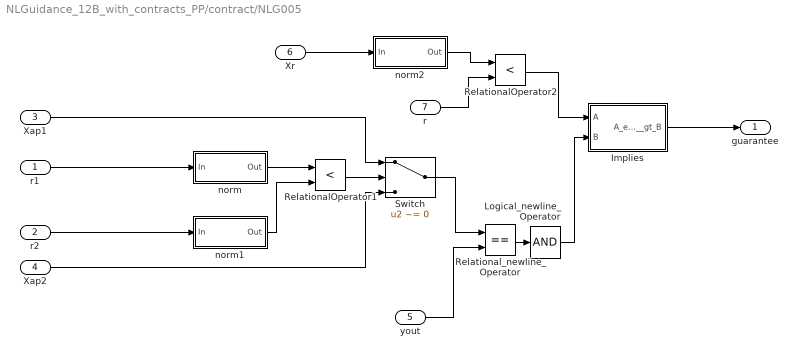
== system NLGuidance_12B_with_contracts_PP/contract/NLG005 ==
  r1 : Inport
  r2 : Inport  Port=2
  Xap1 : Inport  Port=3
  Xap2 : Inport  Port=4
  yout : Inport  Port=5
  Xr : Inport  Port=6
  r : Inport  Port=7
  Implies : Subsystem  AncestorBlock=sldvlib/Verification Utilities/Implies  TreatAsAtomicUnit=on  mask(Design Verifier Implies){}
      mask help: Sldv:shared:sldvlibrary:DVImpliesDesc
      mask Help: helpview(fullfile(docroot,'toolbox','sldv','sldv.map'),'implies')
      mask Display: disp(' ')
  Logical_newline_Operator : Logic  Inputs=1  AllPortsSameDT=off  OutDataTypeStr=boolean
  RelationalOperator1 : RelationalOperator  Operator=<  OutDataTypeStr=boolean  RndMeth=Nearest
  RelationalOperator2 : RelationalOperator  Operator=<  OutDataTypeStr=boolean  RndMeth=Nearest
  Relational_newline_Operator : RelationalOperator  Operator===  OutDataTypeStr=boolean  RndMeth=Simplest
  Switch : Switch  Criteria=u2 ~= 0
  norm : Subsystem  TreatAsAtomicUnit=on
  norm1 : Subsystem  TreatAsAtomicUnit=on
  norm2 : Subsystem  TreatAsAtomicUnit=on
  guarantee : Outport  OutDataTypeStr=boolean  VectorParamsAs1DForOutWhenUnconnected=off
  wires:
  norm/1(Out) -> RelationalOperator1/1
  norm1/1(Out) -> RelationalOperator1/2
  r1/1 -> norm/1(In)
  r2/1 -> norm1/1(In)
  RelationalOperator1/1 -> Switch/2
  Xap1/1 -> Switch/1
  Xap2/1 -> Switch/3
  Switch/1 -> Relational_newline_Operator/1
  yout/1 -> Relational_newline_Operator/2
  Relational_newline_Operator/1 -> Logical_newline_Operator/1
  Logical_newline_Operator/1 -> Implies/2(B)
  Implies/1(A_equal__equal__gt_B) -> guarantee/1
  Xr/1 -> norm2/1(In)
  norm2/1(Out) -> RelationalOperator2/1
  r/1 -> RelationalOperator2/2
  RelationalOperator2/1 -> Implies/1(A)

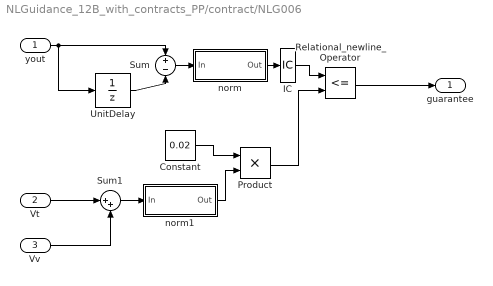
== system NLGuidance_12B_with_contracts_PP/contract/NLG006 ==
  yout : Inport
  Vt : Inport  Port=2
  Vv : Inport  Port=3
  Constant : Constant  Value=0.02  SampleTime=-1
  IC : InitialCondition  Value=0
  Product : Product
  Relational_newline_Operator : RelationalOperator  Operator=<=  OutDataTypeStr=boolean  RndMeth=Simplest
  Sum : Sum  Inputs=+-
  Sum1 : Sum  Inputs=|++
  UnitDelay : UnitDelay  SampleTime=-1  HasFrameUpgradeWarning=on
  norm : Subsystem  TreatAsAtomicUnit=on
  norm1 : Subsystem  TreatAsAtomicUnit=on
  guarantee : Outport  OutDataTypeStr=boolean  VectorParamsAs1DForOutWhenUnconnected=off
  wires:
  yout/1 -> UnitDelay/1, Sum/1
  UnitDelay/1 -> Sum/2
  Sum/1 -> norm/1(In)
  norm/1(Out) -> IC/1
  Constant/1 -> Product/1
  norm1/1(Out) -> Product/2
  Sum1/1 -> norm1/1(In)
  Vt/1 -> Sum1/1
  Vv/1 -> Sum1/2
  Product/1 -> Relational_newline_Operator/2
  Relational_newline_Operator/1 -> guarantee/1
  IC/1 -> Relational_newline_Operator/1

== system NLGuidance_12B_with_contracts_PP/contract/NLG007 ==
  yout : Inport
  Xtarget : Inport  Port=2
  Compare To Zero : Subsystem  AncestorBlock=|  TreatAsAtomicUnit=on  mask(Compare To Zero){relop===, OutDataTypeStr=boolean, ZeroCross=on}
      | simulink/Logic and Bit
      | Operations/Compare
      | To Zero
      mask prompts: relop "Simulink:masks:Operator_MP"; OutDataTypeStr "Simulink:masks:OutputDataType_MP"; ZeroCross "Simulink:masks:EnableZerocrossingDetection_MP"
      mask help: Simulink:masks:CompareToZero_MD
      mask init: same as NLGuidance_12B_with_contracts_PP/contract/NLG002_NLG003/Compare To Zero
      mask TypeOptions relop: == | ~= | < | <= | >= | >
      mask TypeOptions OutDataTypeStr: Simulink:masks:uint8 | Simulink:masks:boolean
      mask Callback ZeroCross: sl('zeroCrossEnable', gcbh);
      mask Display: disp([relop,' 0'])
  Selector : Selector  InputPortWidth=3  IndexOptions=Index vector (dialog)  Indices=3  OutputSizes=1
  Sum : Sum  Inputs=|+-
  guarantee : Outport  OutDataTypeStr=boolean  VectorParamsAs1DForOutWhenUnconnected=off
  wires:
  Compare To Zero/1(y) -> guarantee/1
  Sum/1 -> Selector/1
  yout/1 -> Sum/1
  Xtarget/1 -> Sum/2
  Selector/1 -> Compare To Zero/1(u)

== system NLGuidance_12B_with_contracts_PP/contract/NLG_001 ==
  Vv : Inport
  yout : Inport  Port=2
  Compare To Zero : Subsystem  AncestorBlock=|  TreatAsAtomicUnit=on  mask(Compare To Zero){relop=>, OutDataTypeStr=boolean, ZeroCross=on}
      | simulink/Logic and Bit
      | Operations/Compare
      | To Zero
      mask prompts: relop "Simulink:masks:Operator_MP"; OutDataTypeStr "Simulink:masks:OutputDataType_MP"; ZeroCross "Simulink:masks:EnableZerocrossingDetection_MP"
      mask help: Simulink:masks:CompareToZero_MD
      mask init: same as NLGuidance_12B_with_contracts_PP/contract/NLG002_NLG003/Compare To Zero
      mask TypeOptions relop: == | ~= | < | <= | >= | >
      mask TypeOptions OutDataTypeStr: Simulink:masks:uint8 | Simulink:masks:boolean
      mask Callback ZeroCross: sl('zeroCrossEnable', gcbh);
      mask Display: disp([relop,' 0'])
  Product : Product
  Sum : Sum  Inputs=1
  guarantee : Outport  OutDataTypeStr=boolean  VectorParamsAs1DForOutWhenUnconnected=off
  wires:
  Vv/1 -> Product/1
  yout/1 -> Product/2
  Product/1 -> Sum/1
  Sum/1 -> Compare To Zero/1(u)
  Compare To Zero/1(y) -> guarantee/1

== system NLGuidance_12B_with_contracts_PP/contract/assumeVvnotnull ==
  Vv : Inport
  Compare To Zero : Subsystem  AncestorBlock=|  TreatAsAtomicUnit=on  mask(Compare To Zero){relop=~=, OutDataTypeStr=boolean, ZeroCross=on}
      | simulink/Logic and Bit
      | Operations/Compare
      | To Zero
      mask prompts: relop "Simulink:masks:Operator_MP"; OutDataTypeStr "Simulink:masks:OutputDataType_MP"; ZeroCross "Simulink:masks:EnableZerocrossingDetection_MP"
      mask help: Simulink:masks:CompareToZero_MD
      mask init: same as NLGuidance_12B_with_contracts_PP/contract/NLG002_NLG003/Compare To Zero
      mask TypeOptions relop: == | ~= | < | <= | >= | >
      mask TypeOptions OutDataTypeStr: Simulink:masks:uint8 | Simulink:masks:boolean
      mask Callback ZeroCross: sl('zeroCrossEnable', gcbh);
      mask Display: disp([relop,' 0'])
  all : Logic  Inputs=1  AllPortsSameDT=off  OutDataTypeStr=boolean
  assume : Outport  OutDataTypeStr=boolean  VectorParamsAs1DForOutWhenUnconnected=off
  wires:
  all/1 -> assume/1
  Vv/1 -> Compare To Zero/1(u)
  Compare To Zero/1(y) -> all/1

== system NLGuidance_12B_with_contracts_PP/contract/assumeXrnotnull ==
  Xr : Inport
  Compare To Zero : Subsystem  AncestorBlock=|  TreatAsAtomicUnit=on  mask(Compare To Zero){relop=~=, OutDataTypeStr=boolean, ZeroCross=on}
      | simulink/Logic and Bit
      | Operations/Compare
      | To Zero
      mask prompts: relop "Simulink:masks:Operator_MP"; OutDataTypeStr "Simulink:masks:OutputDataType_MP"; ZeroCross "Simulink:masks:EnableZerocrossingDetection_MP"
      mask help: Simulink:masks:CompareToZero_MD
      mask init: same as NLGuidance_12B_with_contracts_PP/contract/NLG002_NLG003/Compare To Zero
      mask TypeOptions relop: == | ~= | < | <= | >= | >
      mask TypeOptions OutDataTypeStr: Simulink:masks:uint8 | Simulink:masks:boolean
      mask Callback ZeroCross: sl('zeroCrossEnable', gcbh);
      mask Display: disp([relop,' 0'])
  all : Logic  Inputs=1  AllPortsSameDT=off  OutDataTypeStr=boolean
  assume : Outport  OutDataTypeStr=boolean  VectorParamsAs1DForOutWhenUnconnected=off
  wires:
  Xr/1 -> Compare To Zero/1(u)
  Compare To Zero/1(y) -> all/1
  all/1 -> assume/1

== system NLGuidance_12B_with_contracts_PP/NLGuidance/Inner/Act1 ==
  cmd1 : Inport
  ActionPort : ActionPort  ActionPortLabel=if(u1)
  yout : Outport  VectorParamsAs1DForOutWhenUnconnected=off
  wires:
  cmd1/1 -> yout/1

== system NLGuidance_12B_with_contracts_PP/NLGuidance/Inner/Act2 ==
  cmd2 : Inport
  ActionPort : ActionPort  ActionPortLabel=else
  yout : Outport  VectorParamsAs1DForOutWhenUnconnected=off
  wires:
  cmd2/1 -> yout/1

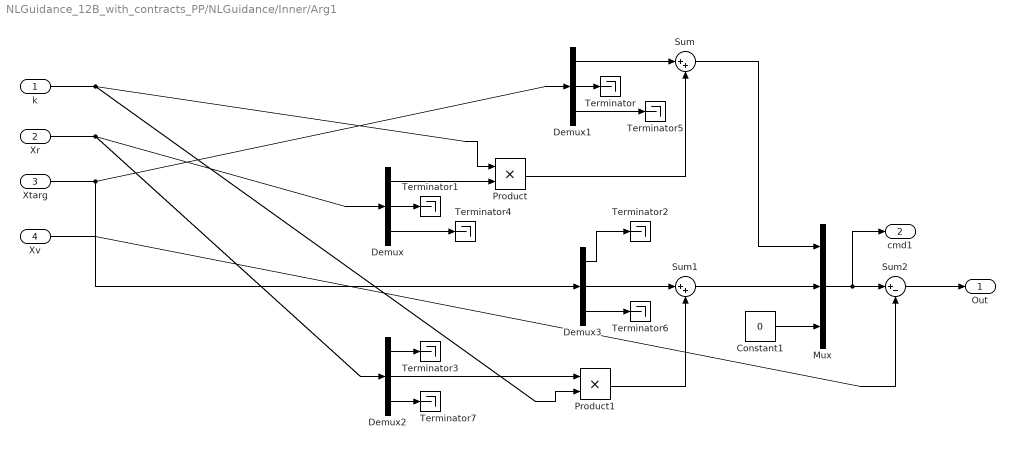
== system NLGuidance_12B_with_contracts_PP/NLGuidance/Inner/Arg1 ==
  k : Inport
  Xr : Inport  Port=2
  Xtarg : Inport  Port=3
  Xv : Inport  Port=4
  Constant1 : Constant  Value=0
  Demux{,1..3} (4 alike) : Demux  Outputs=3
  Mux : Mux  Inputs=3
  Product : Product  RndMeth=Zero
  Product1 : Product  RndMeth=Zero
  Sum : Sum  Inputs=|++
  Sum1 : Sum  Inputs=|++
  Sum2 : Sum  Inputs=|+-
  Terminator{,1..7} (8 alike) : Terminator
  Out : Outport  VectorParamsAs1DForOutWhenUnconnected=off
  cmd1 : Outport  Port=2  VectorParamsAs1DForOutWhenUnconnected=off
  wires:
  Mux/1 -> cmd1/1, Sum2/1
  Demux3/3 -> Terminator6/1
  Demux/2 -> Terminator1/1
  Sum/1 -> Mux/1
  Demux1/2 -> Terminator/1
  Constant1/1 -> Mux/3
  Demux3/2 -> Sum1/1
  Demux2/1 -> Terminator3/1
  Xtarg/1 -> Demux1/1, Demux3/1
  Product/1 -> Sum/2
  k/1 -> Product/1, Product1/2
  Demux/1 -> Product/2
  Xr/1 -> Demux/1, Demux2/1
  Sum1/1 -> Mux/2
  Demux1/1 -> Sum/1
  Demux2/3 -> Terminator7/1
  Sum2/1 -> Out/1
  Demux/3 -> Terminator4/1
  Xv/1 -> Sum2/2
  Demux3/1 -> Terminator2/1
  Demux2/2 -> Product1/1
  Product1/1 -> Sum1/2
  Demux1/3 -> Terminator5/1

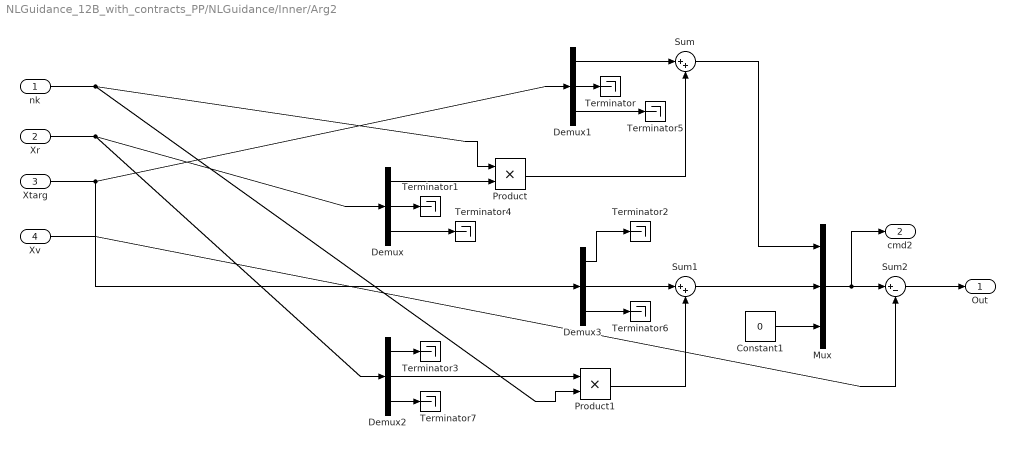
== system NLGuidance_12B_with_contracts_PP/NLGuidance/Inner/Arg2 ==
  nk : Inport
  Xr : Inport  Port=2
  Xtarg : Inport  Port=3
  Xv : Inport  Port=4
  Constant1 : Constant  Value=0
  Demux{,1..3} (4 alike) : Demux  Outputs=3
  Mux : Mux  Inputs=3
  Product : Product  RndMeth=Zero
  Product1 : Product  RndMeth=Zero
  Sum : Sum  Inputs=|++
  Sum1 : Sum  Inputs=|++
  Sum2 : Sum  Inputs=|+-
  Terminator{,1..7} (8 alike) : Terminator
  Out : Outport  VectorParamsAs1DForOutWhenUnconnected=off
  cmd2 : Outport  Port=2  VectorParamsAs1DForOutWhenUnconnected=off
  wires:
  Demux1/3 -> Terminator5/1
  Product1/1 -> Sum1/2
  Demux2/2 -> Product1/1
  Demux3/1 -> Terminator2/1
  Xv/1 -> Sum2/2
  Demux/3 -> Terminator4/1
  Sum2/1 -> Out/1
  Demux2/3 -> Terminator7/1
  Demux1/1 -> Sum/1
  Sum1/1 -> Mux/2
  Xr/1 -> Demux/1, Demux2/1
  Demux/1 -> Product/2
  nk/1 -> Product/1, Product1/2
  Product/1 -> Sum/2
  Xtarg/1 -> Demux1/1, Demux3/1
  Demux2/1 -> Terminator3/1
  Demux3/2 -> Sum1/1
  Constant1/1 -> Mux/3
  Demux1/2 -> Terminator/1
  Sum/1 -> Mux/1
  Demux/2 -> Terminator1/1
  Demux3/3 -> Terminator6/1
  Mux/1 -> cmd2/1, Sum2/1

== system NLGuidance_12B_with_contracts_PP/NLGuidance/Inner/norm ==
  In : Inport
  Math_newline_Function : Math  Operator=square  SaturateOnIntegerOverflow=on
  Math_newline_Function1 : Math  Operator=sqrt  SaturateOnIntegerOverflow=on
  Sumof_newline_Elements : Sum  Inputs=+
  Out : Outport  VectorParamsAs1DForOutWhenUnconnected=off
  wires:
  Math_newline_Function1/1 -> Out/1
  In/1 -> Math_newline_Function/1
  Sumof_newline_Elements/1 -> Math_newline_Function1/1
  Math_newline_Function/1 -> Sumof_newline_Elements/1

== system NLGuidance_12B_with_contracts_PP/NLGuidance/Inner/norm1 ==
  In : Inport
  Math_newline_Function : Math  Operator=square  SaturateOnIntegerOverflow=on
  Math_newline_Function1 : Math  Operator=sqrt  SaturateOnIntegerOverflow=on
  Sumof_newline_Elements : Sum  Inputs=+
  Out : Outport  VectorParamsAs1DForOutWhenUnconnected=off
  wires:
  Math_newline_Function/1 -> Sumof_newline_Elements/1
  Sumof_newline_Elements/1 -> Math_newline_Function1/1
  In/1 -> Math_newline_Function/1
  Math_newline_Function1/1 -> Out/1

== system NLGuidance_12B_with_contracts_PP/NLGuidance/Outer/CCW ==
  Xap1 : Inport
  ActionPort : ActionPort  ActionPortLabel=else
  yout : Outport  VectorParamsAs1DForOutWhenUnconnected=off
  wires:
  Xap1/1 -> yout/1

== system NLGuidance_12B_with_contracts_PP/NLGuidance/Outer/CW ==
  Xap1 : Inport
  ActionPort : ActionPort  ActionPortLabel=if(u1)
  yout : Outport  VectorParamsAs1DForOutWhenUnconnected=off
  wires:
  Xap1/1 -> yout/1

== system NLGuidance_12B_with_contracts_PP/NLGuidance/Outer/cross ==
  A : Inport
  B : Inport  Port=2
  Subsystem1 : Subsystem  TreatAsAtomicUnit=on
  Subsystem2 : Subsystem  TreatAsAtomicUnit=on
  Sum : Sum  Inputs=+|-  SaturateOnIntegerOverflow=on  InputSameDT=on  OutDataTypeStr=Inherit: Same as first input
  C : Outport  VectorParamsAs1DForOutWhenUnconnected=off
  wires:
  B/1 -> Subsystem2/2(B1), Subsystem1/2(B1)
  A/1 -> Subsystem2/1(A1), Subsystem1/1(A1)
  Subsystem2/1(Out1) -> Sum/1
  Sum/1 -> C/1
  Subsystem1/1(Out1) -> Sum/2

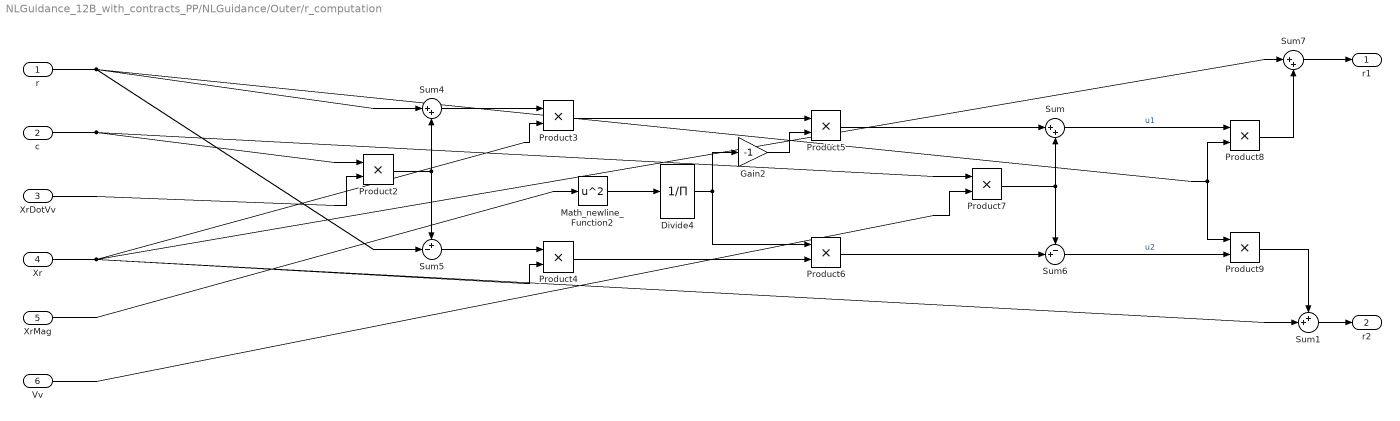
== system NLGuidance_12B_with_contracts_PP/NLGuidance/Outer/r_computation ==
  r : Inport
  c : Inport  Port=2
  XrDotVv : Inport  Port=3
  Xr : Inport  Port=4
  XrMag : Inport  Port=5
  Vv : Inport  Port=6
  Divide4 : Product  Inputs=/
  Gain2 : Gain  Gain=-1
  Math_newline_Function2 : Math  Operator=square  SaturateOnIntegerOverflow=on
  Product{2..9} (8 alike) : Product
  Sum : Sum  Inputs=|++
  Sum1 : Sum  Inputs=++|
  Sum4 : Sum  Inputs=|++
  Sum5 : Sum  Inputs=+-|
  Sum6 : Sum  Inputs=-+|
  Sum7 : Sum  Inputs=|++
  r1 : Outport  VectorParamsAs1DForOutWhenUnconnected=off
  r2 : Outport  Port=2  VectorParamsAs1DForOutWhenUnconnected=off
  wires:
  r/1 -> Sum4/1, Sum5/2, Product9/1, Product8/2
  Sum6/1 -> Product9/2  "u2"
  Gain2/1 -> Product5/2
  Product4/1 -> Product6/2
  XrDotVv/1 -> Product2/2
  Product3/1 -> Product5/1
  Divide4/1 -> Product6/1, Gain2/1
  Sum5/1 -> Product4/1
  Vv/1 -> Product7/2
  Product7/1 -> Sum/2, Sum6/1
  Product8/1 -> Sum7/2
  Sum7/1 -> r1/1
  Product6/1 -> Sum6/2
  Product5/1 -> Sum/1
  Math_newline_Function2/1 -> Divide4/1
  XrMag/1 -> Math_newline_Function2/1
  c/1 -> Product2/1, Product7/1
  Sum4/1 -> Product3/1
  Sum/1 -> Product8/1  "u1"
  Product2/1 -> Sum5/1, Sum4/2
  Product9/1 -> Sum1/1
  Xr/1 -> Sum1/2, Product3/2, Product4/2, Sum7/1
  Sum1/1 -> r2/1

== system NLGuidance_12B_with_contracts_PP/contract/NLG002_NLG003/Compare To Zero ==
  u : Inport
  Compare : RelationalOperator  Operator===  OutDataTypeStr=boolean  RndMeth=Nearest  InputSameDT=on
  Constant : Constant  DisableCoverage=on  Value=0  OutDataTypeStr=Inherit: Inherit via back propagation  PreserveConstantTs=on
  y : Outport
  wires:
  Constant/1 -> Compare/2
  u/1 -> Compare/1
  Compare/1 -> y/1

== system NLGuidance_12B_with_contracts_PP/contract/NLG002_NLG003/DotProduct ==
  In1 : Inport
  In2 : Inport  Port=2
  Product : Product  InputSameDT=on
  SSpec1 : SignalSpecification  Dimensions=3
  SSpec2 : SignalSpecification  Dimensions=3
  Sum : Sum  Inputs=1
  Out1 : Outport  VectorParamsAs1DForOutWhenUnconnected=off
  wires:
  SSpec2/1 -> Product/2
  SSpec1/1 -> Product/1
  Sum/1 -> Out1/1
  Product/1 -> Sum/1
  In1/1 -> SSpec1/1
  In2/1 -> SSpec2/1

== system NLGuidance_12B_with_contracts_PP/contract/NLG002_NLG003/norm1 ==
  In : Inport
  Math_newline_Function : Math  Operator=square  SaturateOnIntegerOverflow=on
  Math_newline_Function1 : Math  Operator=sqrt  SaturateOnIntegerOverflow=on
  Sumof_newline_Elements : Sum  Inputs=+
  Out : Outport  VectorParamsAs1DForOutWhenUnconnected=off
  wires:
  Math_newline_Function/1 -> Sumof_newline_Elements/1
  Sumof_newline_Elements/1 -> Math_newline_Function1/1
  In/1 -> Math_newline_Function/1
  Math_newline_Function1/1 -> Out/1

== system NLGuidance_12B_with_contracts_PP/contract/NLG004/Compare To Zero ==
  u : Inport
  Compare : RelationalOperator  Operator=>  OutDataTypeStr=boolean  RndMeth=Nearest  InputSameDT=on
  Constant : Constant  DisableCoverage=on  Value=0  OutDataTypeStr=Inherit: Inherit via back propagation  PreserveConstantTs=on
  y : Outport
  wires:
  Constant/1 -> Compare/2
  u/1 -> Compare/1
  Compare/1 -> y/1

== system NLGuidance_12B_with_contracts_PP/contract/NLG004/DotProduct ==
  In1 : Inport
  In2 : Inport  Port=2
  Product : Product  InputSameDT=on
  SSpec1 : SignalSpecification  Dimensions=3
  SSpec2 : SignalSpecification  Dimensions=3
  Sum : Sum  Inputs=1
  Out1 : Outport  VectorParamsAs1DForOutWhenUnconnected=off
  wires:
  SSpec2/1 -> Product/2
  SSpec1/1 -> Product/1
  Sum/1 -> Out1/1
  Product/1 -> Sum/1
  In1/1 -> SSpec1/1
  In2/1 -> SSpec2/1

== system NLGuidance_12B_with_contracts_PP/contract/NLG005/Implies ==
  A : Inport
  B : Inport  Port=2
  Logical_newline_Operator : Logic  Operator=OR  AllPortsSameDT=off  OutDataTypeStr=boolean
  Logical_newline_Operator1 : Logic  Operator=NOT  AllPortsSameDT=off  OutDataTypeStr=boolean
  A_equal__equal__gt_B : Outport
  wires:
  Logical_newline_Operator1/1 -> Logical_newline_Operator/1
  A/1 -> Logical_newline_Operator1/1
  Logical_newline_Operator/1 -> A_equal__equal__gt_B/1
  B/1 -> Logical_newline_Operator/2

== system NLGuidance_12B_with_contracts_PP/contract/NLG005/norm ==
  In : Inport
  Math_newline_Function : Math  Operator=square  SaturateOnIntegerOverflow=on
  Math_newline_Function1 : Math  Operator=sqrt  SaturateOnIntegerOverflow=on
  Sumof_newline_Elements : Sum  Inputs=+
  Out : Outport  VectorParamsAs1DForOutWhenUnconnected=off
  wires:
  Math_newline_Function1/1 -> Out/1
  In/1 -> Math_newline_Function/1
  Sumof_newline_Elements/1 -> Math_newline_Function1/1
  Math_newline_Function/1 -> Sumof_newline_Elements/1

== system NLGuidance_12B_with_contracts_PP/contract/NLG005/norm1 ==
  In : Inport
  Math_newline_Function : Math  Operator=square  SaturateOnIntegerOverflow=on
  Math_newline_Function1 : Math  Operator=sqrt  SaturateOnIntegerOverflow=on
  Sumof_newline_Elements : Sum  Inputs=+
  Out : Outport  VectorParamsAs1DForOutWhenUnconnected=off
  wires:
  Math_newline_Function/1 -> Sumof_newline_Elements/1
  Sumof_newline_Elements/1 -> Math_newline_Function1/1
  In/1 -> Math_newline_Function/1
  Math_newline_Function1/1 -> Out/1

== system NLGuidance_12B_with_contracts_PP/contract/NLG005/norm2 ==
  In : Inport
  Math_newline_Function : Math  Operator=square  SaturateOnIntegerOverflow=on
  Math_newline_Function1 : Math  Operator=sqrt  SaturateOnIntegerOverflow=on
  Sumof_newline_Elements : Sum  Inputs=+
  Out : Outport  VectorParamsAs1DForOutWhenUnconnected=off
  wires:
  Math_newline_Function1/1 -> Out/1
  In/1 -> Math_newline_Function/1
  Sumof_newline_Elements/1 -> Math_newline_Function1/1
  Math_newline_Function/1 -> Sumof_newline_Elements/1

== system NLGuidance_12B_with_contracts_PP/contract/NLG006/norm ==
  In : Inport
  Math_newline_Function : Math  Operator=square  SaturateOnIntegerOverflow=on
  Math_newline_Function1 : Math  Operator=sqrt  SaturateOnIntegerOverflow=on
  Sumof_newline_Elements : Sum  Inputs=+
  Out : Outport  VectorParamsAs1DForOutWhenUnconnected=off
  wires:
  Math_newline_Function1/1 -> Out/1
  In/1 -> Math_newline_Function/1
  Sumof_newline_Elements/1 -> Math_newline_Function1/1
  Math_newline_Function/1 -> Sumof_newline_Elements/1

== system NLGuidance_12B_with_contracts_PP/contract/NLG006/norm1 ==
  In : Inport
  Math_newline_Function : Math  Operator=square  SaturateOnIntegerOverflow=on
  Math_newline_Function1 : Math  Operator=sqrt  SaturateOnIntegerOverflow=on
  Sumof_newline_Elements : Sum  Inputs=+
  Out : Outport  VectorParamsAs1DForOutWhenUnconnected=off
  wires:
  Math_newline_Function1/1 -> Out/1
  In/1 -> Math_newline_Function/1
  Sumof_newline_Elements/1 -> Math_newline_Function1/1
  Math_newline_Function/1 -> Sumof_newline_Elements/1

== system NLGuidance_12B_with_contracts_PP/contract/NLG007/Compare To Zero ==
  u : Inport
  Compare : RelationalOperator  Operator===  OutDataTypeStr=boolean  RndMeth=Nearest  InputSameDT=on
  Constant : Constant  DisableCoverage=on  Value=0  OutDataTypeStr=Inherit: Inherit via back propagation  PreserveConstantTs=on
  y : Outport
  wires:
  Constant/1 -> Compare/2
  u/1 -> Compare/1
  Compare/1 -> y/1

== system NLGuidance_12B_with_contracts_PP/contract/NLG_001/Compare To Zero ==
  u : Inport
  Compare : RelationalOperator  Operator=>  OutDataTypeStr=boolean  RndMeth=Nearest  InputSameDT=on
  Constant : Constant  DisableCoverage=on  Value=0  OutDataTypeStr=Inherit: Inherit via back propagation  PreserveConstantTs=on
  y : Outport
  wires:
  Constant/1 -> Compare/2
  u/1 -> Compare/1
  Compare/1 -> y/1

== system NLGuidance_12B_with_contracts_PP/contract/assumeVvnotnull/Compare To Zero ==
  u : Inport
  Compare : RelationalOperator  Operator=~=  OutDataTypeStr=boolean  RndMeth=Nearest  InputSameDT=on
  Constant : Constant  DisableCoverage=on  Value=0  OutDataTypeStr=Inherit: Inherit via back propagation  PreserveConstantTs=on
  y : Outport
  wires:
  Constant/1 -> Compare/2
  u/1 -> Compare/1
  Compare/1 -> y/1

== system NLGuidance_12B_with_contracts_PP/contract/assumeXrnotnull/Compare To Zero ==
  u : Inport
  Compare : RelationalOperator  Operator=~=  OutDataTypeStr=boolean  RndMeth=Nearest  InputSameDT=on
  Constant : Constant  DisableCoverage=on  Value=0  OutDataTypeStr=Inherit: Inherit via back propagation  PreserveConstantTs=on
  y : Outport
  wires:
  Constant/1 -> Compare/2
  u/1 -> Compare/1
  Compare/1 -> y/1

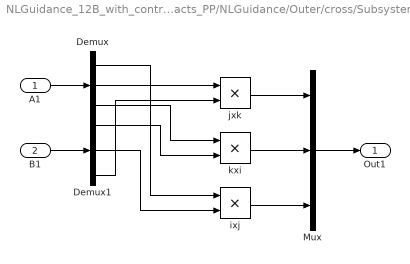
== system NLGuidance_12B_with_contracts_PP/NLGuidance/Outer/cross/Subsystem1 ==
  A1 : Inport
  B1 : Inport  Port=2
  Demux : Demux  Outputs=3
  Demux1 : Demux  Outputs=3
  Mux : Mux  Inputs=3
  ixj : Product  SaturateOnIntegerOverflow=on  InputSameDT=on  OutDataTypeStr=Inherit: Same as first input
  jxk : Product  SaturateOnIntegerOverflow=on  InputSameDT=on  OutDataTypeStr=Inherit: Same as first input
  kxi : Product  SaturateOnIntegerOverflow=on  InputSameDT=on  OutDataTypeStr=Inherit: Same as first input
  Out1 : Outport  VectorParamsAs1DForOutWhenUnconnected=off
  wires:
  Demux/2 -> jxk/1
  Demux1/3 -> jxk/2
  A1/1 -> Demux/1
  Demux/3 -> kxi/1
  Mux/1 -> Out1/1
  jxk/1 -> Mux/1
  B1/1 -> Demux1/1
  kxi/1 -> Mux/2
  Demux1/2 -> ixj/2
  ixj/1 -> Mux/3
  Demux/1 -> ixj/1
  Demux1/1 -> kxi/2

== system NLGuidance_12B_with_contracts_PP/NLGuidance/Outer/cross/Subsystem2 ==
  A1 : Inport
  B1 : Inport  Port=2
  Demux : Demux  Outputs=3
  Demux1 : Demux  Outputs=3
  Mux : Mux  Inputs=3
  ixj : Product  SaturateOnIntegerOverflow=on  InputSameDT=on  OutDataTypeStr=Inherit: Same as first input
  jxk : Product  SaturateOnIntegerOverflow=on  InputSameDT=on  OutDataTypeStr=Inherit: Same as first input
  kxi : Product  SaturateOnIntegerOverflow=on  InputSameDT=on  OutDataTypeStr=Inherit: Same as first input
  Out1 : Outport  VectorParamsAs1DForOutWhenUnconnected=off
  wires:
  Demux1/1 -> kxi/2
  Demux/1 -> ixj/1
  ixj/1 -> Mux/3
  Demux1/2 -> ixj/2
  kxi/1 -> Mux/2
  B1/1 -> Demux1/1
  jxk/1 -> Mux/1
  Mux/1 -> Out1/1
  Demux/3 -> kxi/1
  A1/1 -> Demux/1
  Demux1/3 -> jxk/2
  Demux/2 -> jxk/1
